simulink subsystem "rss_ShOffFlgConfSenl"  (R2023a)
settings: Solver=VariableStepAuto  StartTime=0.0  StopTime=10.0  RelTol=1e-3
undefined symbols (not defined in the file): ENM_SYS_STATUS
libraries: simulink x3
settings Model: Creator=xiaoqiang.yuan  LastModifiedBy=xiaoqiang.yuan

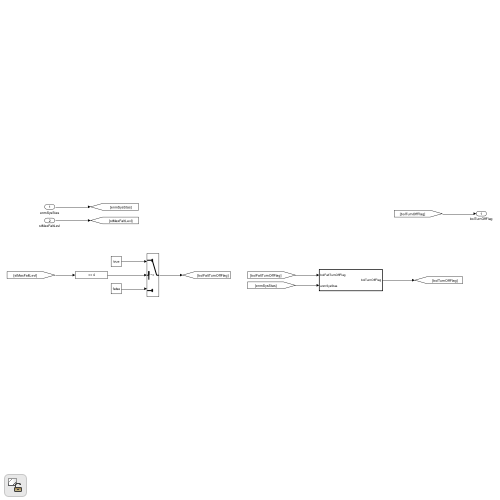
[thumbnail: Simulink's stored preview of the top-level diagram]
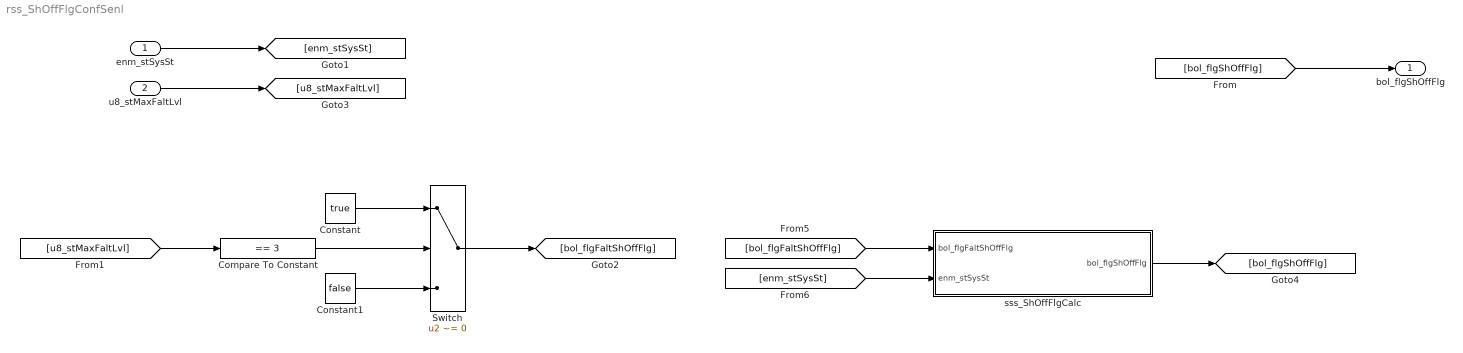
== system rss_ShOffFlgConfSenl ==
  enm_stSysSt : Inport  OutDataTypeStr=Enum: ENM_SYS_STATUS
  u8_stMaxFaltLvl : Inport  Port=2  OutDataTypeStr=uint8
  Compare To Constant : simulink/Logic and Bit Operations/Compare To Constant  relop===  const=3  OutDataTypeStr=boolean
  Constant : Constant  Value=true  OutDataTypeStr=boolean
  Constant1 : Constant  Value=false  OutDataTypeStr=boolean
  Switch : Switch  Criteria=u2 ~= 0  SaturateOnIntegerOverflow=off  InputSameDT=off
  sss_ShOffFlgCalc : Subsystem
  bol_flgShOffFlg : Outport
  wires:
  [enm_stSysSt] -> sss_ShOffFlgCalc/2(enm_stSysSt)
  [bol_flgFaltShOffFlg] -> sss_ShOffFlgCalc/1(bol_flgFaltShOffFlg)
  sss_ShOffFlgCalc/1(bol_flgShOffFlg) -> [bol_flgShOffFlg]
  [bol_flgShOffFlg] -> bol_flgShOffFlg/1
  enm_stSysSt/1 -> [enm_stSysSt]
  u8_stMaxFaltLvl/1 -> [u8_stMaxFaltLvl]
  Constant1/1 -> Switch/3
  Switch/1 -> [bol_flgFaltShOffFlg]
  Constant/1 -> Switch/1
  [u8_stMaxFaltLvl] -> Compare To Constant/1
  Compare To Constant/1 -> Switch/2

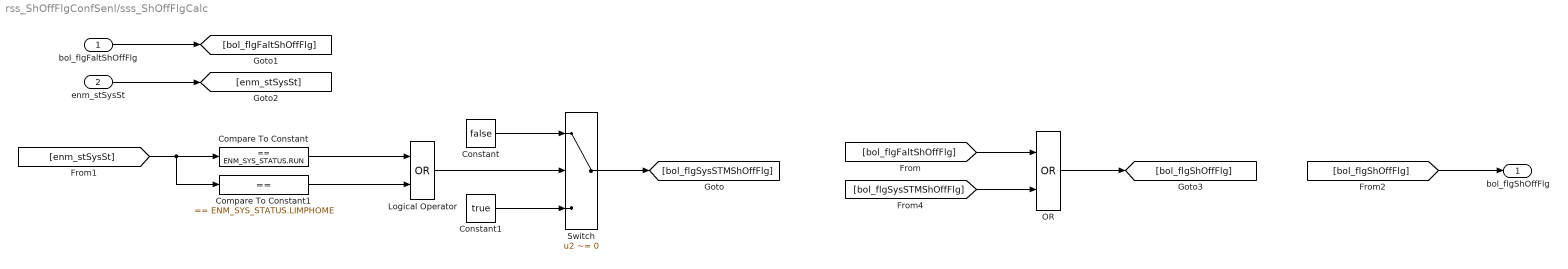
== system rss_ShOffFlgConfSenl/sss_ShOffFlgCalc ==
  bol_flgFaltShOffFlg : Inport
  enm_stSysSt : Inport  Port=2
  Compare To Constant : simulink/Logic and Bit Operations/Compare To Constant  relop===  const=ENM_SYS_STATUS.RUN  OutDataTypeStr=boolean
  Compare To Constant1 : simulink/Logic and Bit Operations/Compare To Constant  relop===  const=ENM_SYS_STATUS.LIMPHOME  OutDataTypeStr=boolean
  Constant : Constant  Value=false  OutDataTypeStr=boolean
  Constant1 : Constant  Value=true  OutDataTypeStr=boolean
  Logical Operator : Logic  Operator=OR  AllPortsSameDT=off  OutDataTypeStr=boolean
  OR : Logic  Operator=OR  AllPortsSameDT=off  OutDataTypeStr=boolean
  Switch : Switch  Criteria=u2 ~= 0  SaturateOnIntegerOverflow=off  InputSameDT=off
  bol_flgShOffFlg : Outport
  wires:
  Compare To Constant/1 -> Logical Operator/1
  Compare To Constant1/1 -> Logical Operator/2
  [enm_stSysSt] -> Compare To Constant1/1, Compare To Constant/1
  Logical Operator/1 -> Switch/2
  Constant/1 -> Switch/1
  Constant1/1 -> Switch/3
  Switch/1 -> [bol_flgSysSTMShOffFlg]
  [bol_flgSysSTMShOffFlg] -> OR/2
  bol_flgFaltShOffFlg/1 -> [bol_flgFaltShOffFlg]
  enm_stSysSt/1 -> [enm_stSysSt]
  [bol_flgFaltShOffFlg] -> OR/1
  OR/1 -> [bol_flgShOffFlg]
  [bol_flgShOffFlg] -> bol_flgShOffFlg/1
